simulink model "tubemodel"  (Simulink 7.3)
settings: Solver=FixedStepDiscrete  StartTime=0.0  StopTime=1  FixedStep=1/10000  MaxStep=1/11025  MinStep=1/11025  RelTol=1e-3
libraries: simulink x1
settings Model: Creator=Hörnstein  LastModifiedBy=jonas
settings SolverCC: InitialStep=1/11025
settings OptimizationCC: InitFltsAndDblsToZero=on
settings DebuggingCC: AlgebraicLoopMsg=none  SaveWithParameterizedLinksMsg=none  SignalResolutionControl=TryResolveAllWithWarning  MultiTaskDSMMsg=warning  MultiTaskCondExecSysMsg=none
settings RTWCC: IncludeERTFirstTime=on
settings GRTTargetCC: TargetFcnLib=ansi_tfl_tmw.mat

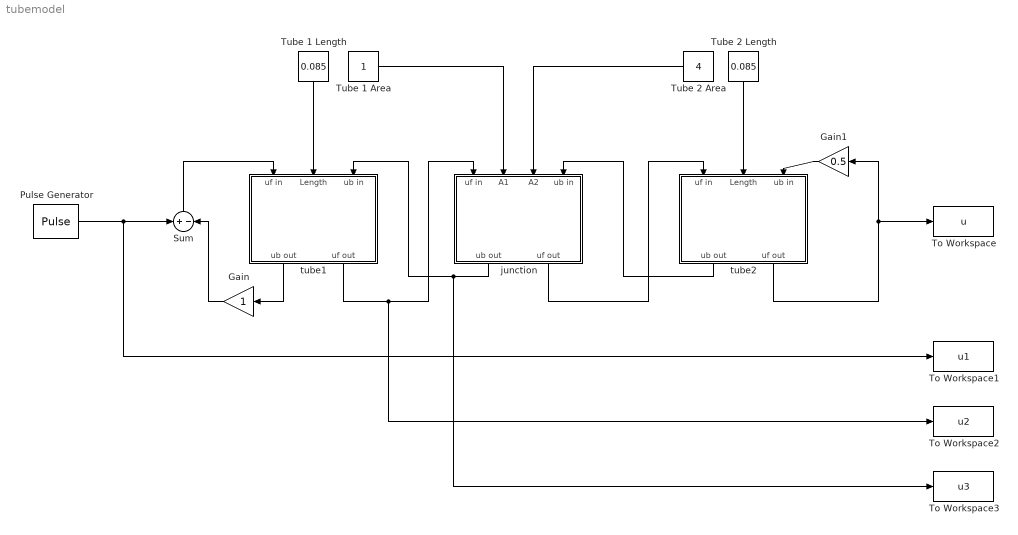
== system tubemodel ==
  Gain : Gain  ParameterDataType=sfix(16)  ParameterScaling=2^0  OutDataType=sfix(16)  OutScaling=2^0
  Gain1 : Gain  Gain=0.5  ParameterDataType=sfix(16)  ParameterScaling=2^0  OutDataType=sfix(16)  OutScaling=2^0
  Pulse Generator : DiscretePulseGenerator  PulseType=Time based  Amplitude=1  Period=0.01  PulseWidth=1  PhaseDelay=0  SampleTime=1
  Sum : Sum  Inputs=+|-  OutDataType=sfix(16)  OutScaling=2^0
  To Workspace : ToWorkspace  VariableName=u  SampleTime=-1  SaveFormat=Array
  To Workspace1 : ToWorkspace  VariableName=u1  SampleTime=-1  SaveFormat=Array
  To Workspace2 : ToWorkspace  VariableName=u2  SampleTime=-1  SaveFormat=Array
  To Workspace3 : ToWorkspace  VariableName=u3  SampleTime=-1  SaveFormat=Array
  Tube 1 Area : Constant  OutDataType=sfix(16)  OutScaling=2^0
  Tube 1 Length : Constant  Value=0.085  OutDataType=sfix(16)  OutScaling=2^0
  Tube 2 Area : Constant  Value=4  OutDataType=sfix(16)  OutScaling=2^0
  Tube 2 Length : Constant  Value=0.085  OutDataType=sfix(16)  OutScaling=2^0
  junction : Subsystem
  tube1 : Subsystem
  tube2 : Subsystem
  wires:
  Tube 1 Area/1 -> junction/2(A1)
  Gain/1 -> Sum/2
  junction/2(uf out) -> tube2/1(uf in)
  tube1/2(uf out) -> junction/1(uf in), To Workspace2/1
  junction/1(ub out) -> tube1/3(ub in), To Workspace3/1
  tube2/1(ub out) -> junction/4(ub in)
  Tube 2 Length/1 -> tube2/2(Length)
  tube2/2(uf out) -> To Workspace/1, Gain1/1
  tube1/1(ub out) -> Gain/1
  Tube 1 Length/1 -> tube1/2(Length)
  Sum/1 -> tube1/1(uf in)
  Tube 2 Area/1 -> junction/3(A2)
  Gain1/1 -> tube2/3(ub in)
  Pulse Generator/1 -> Sum/1, To Workspace1/1

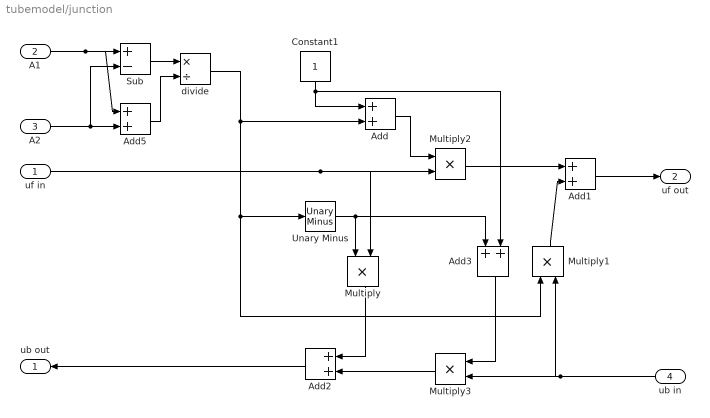
== system tubemodel/junction ==
  uf in : Inport  OutDataType=sfix(16)  OutScaling=2^0
  A1 : Inport  Port=2  OutDataType=sfix(16)  OutScaling=2^0
  A2 : Inport  Port=3  OutDataType=sfix(16)  OutScaling=2^0
  ub in : Inport  Port=4  OutDataType=sfix(16)  OutScaling=2^0
  Add{,1..3,5} (5 alike) : Sum  OutDataType=fixdt(1, 16)  OutScaling=2^-10
  Constant1 : Constant  OutDataType=sfix(16)  OutScaling=2^0
  Multiply{,1..3} (4 alike) : Product  Inputs=**  OutDataType=sfix(16)  OutScaling=2^-10
  Sub : Sum  Inputs=+-  OutDataType=fixdt(1, 16)  OutScaling=2^-10
  Unary Minus : simulink/Math Operations/Unary Minus  DoSatur=off
  divide : Product  Inputs=*/  OutDataType=sfix(16)  OutScaling=2^-10
  ub out : Outport  OutDataType=sfix(16)  OutScaling=2^0
  uf out : Outport  Port=2  OutDataType=sfix(16)  OutScaling=2^0
  wires:
  Add1/1 -> uf out/1
  Unary Minus/1 -> Multiply/1, Add3/1
  Constant1/1 -> Add/1, Add3/2
  Add/1 -> Multiply2/1
  Multiply2/1 -> Add1/1
  Multiply1/1 -> Add1/2
  Multiply/1 -> Add2/1
  Multiply3/1 -> Add2/2
  ub in/1 -> Multiply3/2, Multiply1/2
  Add3/1 -> Multiply3/1
  uf in/1 -> Multiply2/2, Multiply/2
  Add2/1 -> ub out/1
  divide/1 -> Multiply1/1, Unary Minus/1, Add/2
  A1/1 -> Sub/1, Add5/1
  A2/1 -> Sub/2, Add5/2
  Sub/1 -> divide/1
  Add5/1 -> divide/2

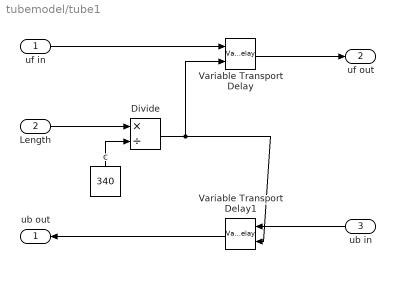
== system tubemodel/tube1 ==
  uf in : Inport  OutDataType=sfix(16)  OutScaling=2^0
  Length : Inport  Port=2  OutDataType=sfix(16)  OutScaling=2^0
  ub in : Inport  Port=3  OutDataType=sfix(16)  OutScaling=2^0
  Divide : Product  Inputs=*/  OutDataType=sfix(16)  OutScaling=2^-10
  Variable Transport Delay : VariableTransportDelay  MaximumDelay=50000  MaximumPoints=50000
  Variable Transport Delay1 : VariableTransportDelay  MaximumDelay=50000  MaximumPoints=50000
  c : Constant  Value=340  OutDataType=sfix(16)  OutScaling=2^0
  ub out : Outport  OutDataType=sfix(16)  OutScaling=2^0
  uf out : Outport  Port=2  OutDataType=sfix(16)  OutScaling=2^0
  wires:
  Variable Transport Delay/1 -> uf out/1
  ub in/1 -> Variable Transport Delay1/1
  Variable Transport Delay1/1 -> ub out/1
  uf in/1 -> Variable Transport Delay/1
  c/1 -> Divide/2
  Length/1 -> Divide/1
  Divide/1 -> Variable Transport Delay/2, Variable Transport Delay1/2

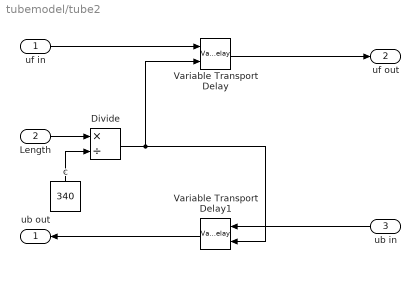
== system tubemodel/tube2 ==
  uf in : Inport  OutDataType=sfix(16)  OutScaling=2^0
  Length : Inport  Port=2  OutDataType=sfix(16)  OutScaling=2^0
  ub in : Inport  Port=3  OutDataType=sfix(16)  OutScaling=2^0
  Divide : Product  Inputs=*/  OutDataType=sfix(16)  OutScaling=2^-10
  Variable Transport Delay : VariableTransportDelay  MaximumDelay=50000  MaximumPoints=50000
  Variable Transport Delay1 : VariableTransportDelay  MaximumDelay=50000  MaximumPoints=50000
  c : Constant  Value=340  OutDataType=sfix(16)  OutScaling=2^0
  ub out : Outport  OutDataType=sfix(16)  OutScaling=2^0
  uf out : Outport  Port=2  OutDataType=sfix(16)  OutScaling=2^0
  wires:
  Variable Transport Delay/1 -> uf out/1
  ub in/1 -> Variable Transport Delay1/1
  Variable Transport Delay1/1 -> ub out/1
  uf in/1 -> Variable Transport Delay/1
  c/1 -> Divide/2
  Length/1 -> Divide/1
  Divide/1 -> Variable Transport Delay/2, Variable Transport Delay1/2
